simulink model "SUBS_ACC_IZAJE"  (R2024b)
settings: Solver=VariableStepAuto  StartTime=0.0  StopTime=10.0  RelTol=1e-3
undefined symbols (not defined in the file): bhd, bhEb, bhm, ih, Jhd_hEb, Jhm_hb, rhd, Thb_Max, ThEb_Max
settings Model: Creator=juani  LastModifiedBy=juani

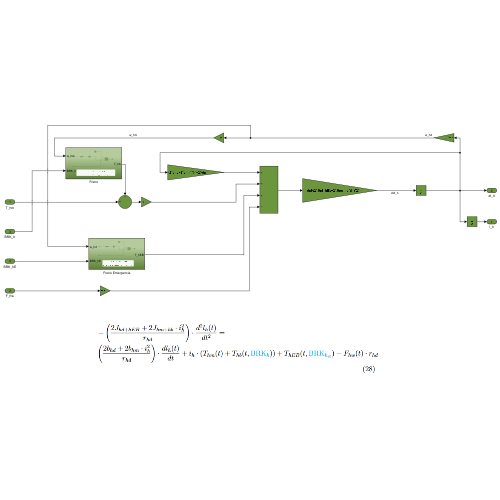
[thumbnail: Simulink's stored preview of the top-level diagram]
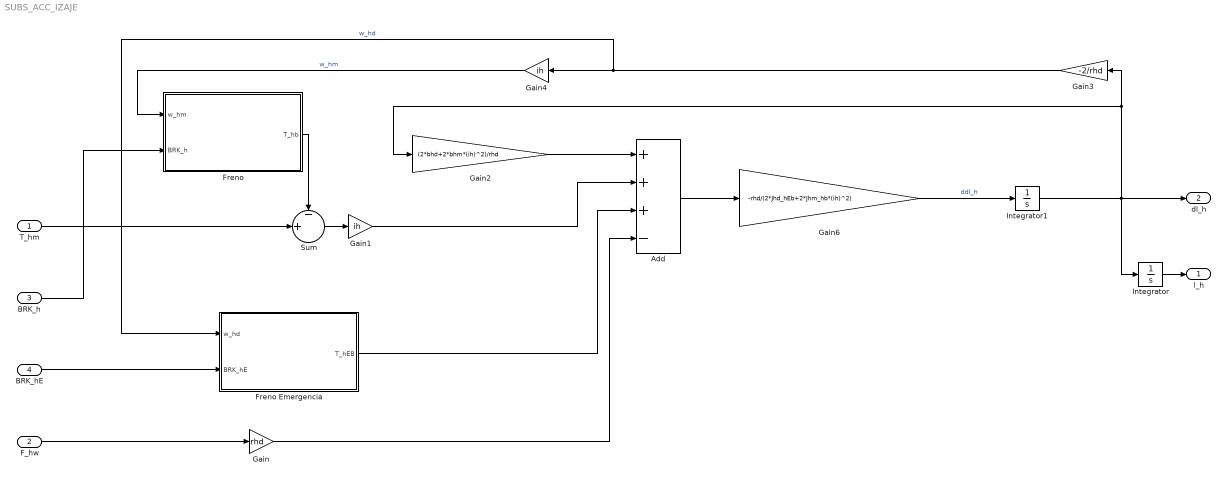
== system SUBS_ACC_IZAJE ==
  T_hm : Inport
  F_hw : Inport  Port=2
  BRK_h : Inport  Port=3
  BRK_hE : Inport  Port=4
  Add : Sum  Inputs=+++-
  Freno : Subsystem
  Freno Emergencia : Subsystem
  Gain : Gain  Gain=rhd
  Gain1 : Gain  Gain=ih
  Gain2 : Gain  Gain=(2*bhd+2*bhm*(ih)^2)/rhd
  Gain3 : Gain  Gain=-2/rhd
  Gain4 : Gain  Gain=ih
  Gain6 : Gain  Gain=-rhd/(2*Jhd_hEb+2*Jhm_hb*(ih)^2)
  Integrator : Integrator
  Integrator1 : Integrator
  Sum : Sum  Inputs=-|+||
  l_h : Outport
  dl_h : Outport  Port=2
  wires:
  F_hw/1 -> Gain/1
  Gain/1 -> Add/4
  Freno Emergencia/1(T_hEB) -> Add/3
  T_hm/1 -> Sum/2
  Sum/1 -> Gain1/1
  Gain1/1 -> Add/2
  Integrator1/1 -> Integrator/1, Gain3/1, Gain2/1, dl_h/1
  Gain2/1 -> Add/1
  Gain3/1 -> Freno Emergencia/1(w_hd), Gain4/1  "w_hd"
  Gain4/1 -> Freno/1(w_hm)  "w_hm"
  Integrator/1 -> l_h/1
  Gain6/1 -> Integrator1/1  "ddl_h"
  Add/1 -> Gain6/1
  BRK_h/1 -> Freno/2(BRK_h)
  Freno/1(T_hb) -> Sum/1
  BRK_hE/1 -> Freno Emergencia/2(BRK_hE)

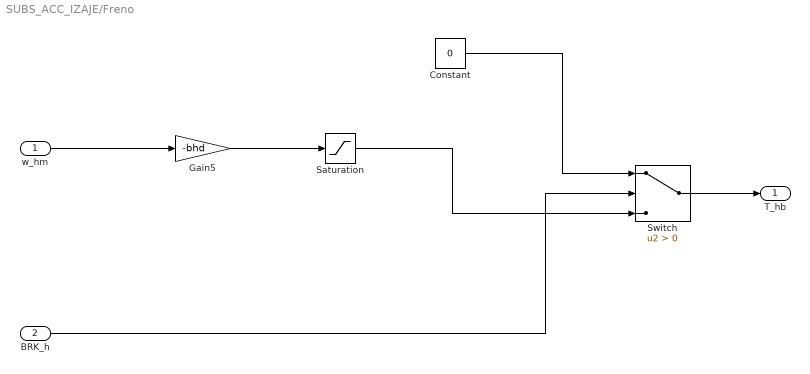
== system SUBS_ACC_IZAJE/Freno ==
  w_hm : Inport
  BRK_h : Inport  Port=2
  Constant : Constant  Value=0
  Gain5 : Gain  Gain=-bhd
  Saturation : Saturate  UpperLimit=Thb_Max  LowerLimit=-Thb_Max
  Switch : Switch  Criteria=u2 > Threshold  SaturateOnIntegerOverflow=off  InputSameDT=off
  T_hb : Outport
  wires:
  Gain5/1 -> Saturation/1
  BRK_h/1 -> Switch/2
  Saturation/1 -> Switch/3
  Constant/1 -> Switch/1
  w_hm/1 -> Gain5/1
  Switch/1 -> T_hb/1

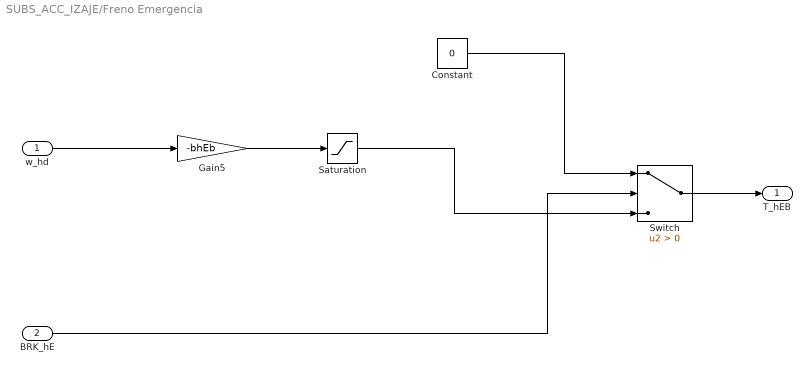
== system SUBS_ACC_IZAJE/Freno Emergencia ==
  w_hd : Inport
  BRK_hE : Inport  Port=2
  Constant : Constant  Value=0
  Gain5 : Gain  Gain=-bhEb
  Saturation : Saturate  UpperLimit=ThEb_Max  LowerLimit=-ThEb_Max
  Switch : Switch  Criteria=u2 > Threshold  SaturateOnIntegerOverflow=off  InputSameDT=off
  T_hEB : Outport
  wires:
  Gain5/1 -> Saturation/1
  BRK_hE/1 -> Switch/2
  Saturation/1 -> Switch/3
  Constant/1 -> Switch/1
  w_hd/1 -> Gain5/1
  Switch/1 -> T_hEB/1
